simulink model "IVR"  (R2017b)
settings: Solver=VariableStepAuto  StartTime=0.0  StopTime=4e-06  MaxStep=1e-09  MinStep=1e-13  RelTol=1e-3
values from neighbouring files (symbols this model uses):
  ADC_reso = (ADC_higher_range-ADC_lower_range)/2^ADC_reso_bits    [ivr_specs_gen.m]
  DPWM_reso = (DPWM_upper_limit-DPWM_lower_limit)/2^DPWM_reso_bits    [ivr_specs_gen.m]
libraries: simulink x1, powerlib_meascontrol x1
settings Model: Creator=ndasari3  LastModifiedBy=nihar
settings CodeAppCC: StateflowObjectComments=on
settings SimscapeCC: SimscapeNormalizeSystem=off

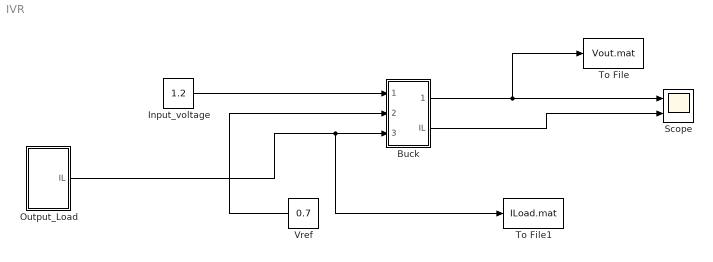
== system IVR ==
  Buck : Subsystem
  Input_voltage : Constant  Value=1.2
  Output_Load : Subsystem
  Scope : Scope  NumInputPorts=2
  To File : ToFile  Filename=Vout.mat  MatrixName=Vout  SaveFormat=Timeseries
  To File1 : ToFile  Filename=ILoad.mat  MatrixName=ILoad  SaveFormat=Timeseries
  Vref : Constant  Value=0.7
  wires:
  Input_voltage/1 -> Buck/1(Vin)
  Vref/1 -> Buck/2(Vref)
  Output_Load/1(IL) -> To File1/1, Buck/3(Iout)
  Buck/1(Vout) -> To File/1, Scope/1
  Buck/2(IL) -> Scope/2

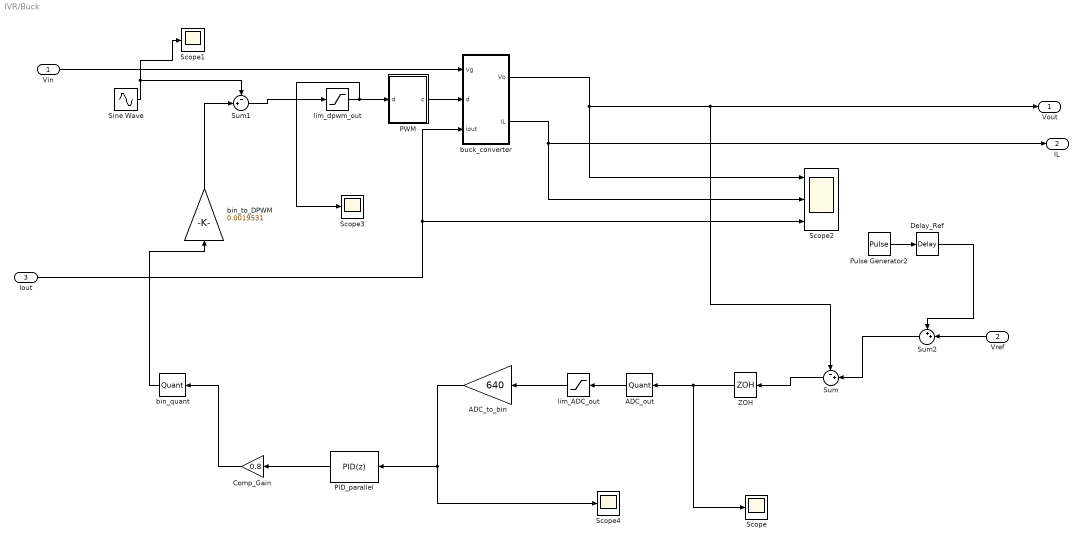
== system IVR/Buck ==
  Vin : Inport
  Vref : Inport  Port=2
  Iout : Inport  Port=3
  ADC_out : Quantizer  QuantizationInterval=0.0015625
  ADC_to_bin : Gain  Gain=640  RndMeth=Nearest
  Comp_Gain : Gain  Gain=0.8
  Delay_Ref : TransportDelay  DelayTime=0  BufferSize=64512
  PID_parallel : simulink/Continuous/PID Controller  Controller=PID  TimeDomain=Discrete-time  SampleTime=4e-09  IntegratorMethod=Backward Euler  FilterMethod=Forward Euler  Form=Parallel  UseFilter=off  ControllerParametersSource=internal  P=1.338  I=10436585.834  D=3.7629e-09  N=100  InitialConditionSource=internal  InitialConditionForIntegrator=0  InitialConditionForFilter=0  ExternalReset=none  LimitOutput=on  UpperSaturationLimit=1/ADC_reso  LowerSaturationLimit=0  LinearizeAsGain=off  AntiWindupMode=none  Kb=1  TrackingMode=off  Kt=1  PParamMin=[]  PParamMax=[]  IParamMin=[]  IParamMax=[]  DParamMin=[]  DParamMax=[]  NParamMin=[]  NParamMax=[]  KbParamMin=[]  KbParamMax=[]  KtParamMin=[]  KtParamMax=[]  POutMin=[]  POutMax=[]  IOutMin=[]  IOutMax=[]  DOutMin=[]  DOutMax=[]  NOutMin=[]  NOutMax=[]  KbOutMin=[]  KbOutMax=[]  KtOutMin=[]  KtOutMax=[]  IntegratorOutMin=[]  IntegratorOutMax=[]  FilterOutMin=[]  FilterOutMax=[]  SumOutMin=[]  SumOutMax=[]  SumI1OutMin=[]  SumI1OutMax=[]  SumI2OutMin=[]  SumI2OutMax=[]  SumI3OutMin=[]  SumI3OutMax=[]  SumDOutMin=[]  SumDOutMax=[]  SaturationOutMin=[]  SaturationOutMax=[]  IntegratorContinuousStateAttributes=''  IntegratorStateMustResolveToSignalObject=off  IntegratorRTWStateStorageClass=Auto  FilterContinuousStateAttributes=''  FilterStateMustResolveToSignalObject=off  FilterRTWStateStorageClass=Auto  DifferentiatorICPrevScaledInput=0  DifferentiatorOutMin=[]  DifferentiatorOutMax=[]  InitialConditionSetting=State (most efficient)  FilterDiffOutCoefMin=[]  FilterDiffOutCoefMax=[]  SumDenOutMin=[]  SumDenOutMax=[]  SumNumOutMin=[]  SumNumOutMax=[]  ReciprocalOutMin=[]  ReciprocalOutMax=[]  DivideOutMin=[]  DivideOutMax=[]  TunerSelectOption=Transfer Function Based (PID Tuner App)
  PWM : Subsystem
  Pulse Generator2 : DiscretePulseGenerator  PulseType=Time based  Amplitude=0  Period=1e-6  PulseWidth=50  PhaseDelay=5e-6
  Scope{,1,3..4} (4 alike) : Scope
  Scope2 : Scope  NumInputPorts=3
  Sine Wave : Sin  SineType=Sample based  Amplitude=DPWM_reso/4  Bias=DPWM_reso/4  Frequency=2*pi*125e6  Samples=3  SampleTime=4e-9
  Sum : Sum  Inputs=-+|  SaturateOnIntegerOverflow=on  InputSameDT=on  OutDataTypeStr=Inherit: Same as first input
  Sum1 : Sum  Inputs=-+|  SaturateOnIntegerOverflow=on  InputSameDT=on  OutDataTypeStr=Inherit: Same as first input
  Sum2 : Sum  Inputs=++|  SaturateOnIntegerOverflow=on  InputSameDT=on  OutDataTypeStr=Inherit: Same as first input
  ZOH : ZeroOrderHold  SampleTime=4e-09
  bin_quant : Quantizer  QuantizationInterval=1
  bin_to_DPWM : Gain  Gain=0.0019531
  buck_converter : Subsystem
  lim_ADC_out : Saturate  UpperLimit=0.2  LowerLimit=-0.2  ZeroCross=off
  lim_dpwm_out : Saturate  UpperLimit=1  LowerLimit=0
  Vout : Outport
  IL : Outport  Port=2
  wires:
  Vin/1 -> buck_converter/1(Vg)
  Vref/1 -> Sum2/2
  Iout/1 -> buck_converter/3(iout), Scope2/3
  Pulse Generator2/1 -> Delay_Ref/1
  Delay_Ref/1 -> Sum2/1
  Sum2/1 -> Sum/2
  Comp_Gain/1 -> bin_quant/1
  ADC_out/1 -> lim_ADC_out/1
  bin_quant/1 -> bin_to_DPWM/1
  lim_ADC_out/1 -> ADC_to_bin/1
  ADC_to_bin/1 -> PID_parallel/1, Scope4/1
  buck_converter/1(Vo) -> Sum/1, Vout/1, Scope2/1
  lim_dpwm_out/1 -> Scope3/1, PWM/1(d)
  Sum/1 -> ZOH/1
  buck_converter/2(IL) -> IL/1, Scope2/2
  ZOH/1 -> Scope/1, ADC_out/1
  bin_to_DPWM/1 -> Sum1/2
  PWM/1(c) -> buck_converter/2(d)
  Sine Wave/1 -> Sum1/1, Scope1/1
  Sum1/1 -> lim_dpwm_out/1
  PID_parallel/1 -> Comp_Gain/1

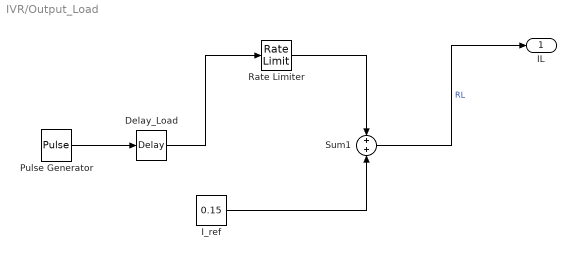
== system IVR/Output_Load ==
  Delay_Load : TransportDelay  DelayTime=2e-06  BufferSize=64512
  I_ref : Constant  Value=0.15
  Pulse Generator : DiscretePulseGenerator  PulseType=Time based  Amplitude=0.25  Period=1  PulseWidth=50
  Rate Limiter : RateLimiter  RisingSlewLimit=1/1e-9  FallingSlewLimit=-1/1e-9  SampleTimeMode=inherited
  Sum1 : Sum  Inputs=+|+  SaturateOnIntegerOverflow=on  InputSameDT=on  OutDataTypeStr=Inherit: Same as first input
  IL : Outport
  wires:
  Delay_Load/1 -> Rate Limiter/1
  Sum1/1 -> IL/1  "RL"
  I_ref/1 -> Sum1/2
  Pulse Generator/1 -> Delay_Load/1
  Rate Limiter/1 -> Sum1/1

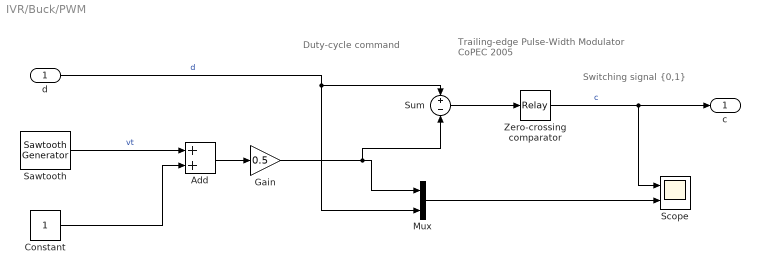
== system IVR/Buck/PWM ==
  note: Duty-cycle
      | command
  note: Switching signal {0,1}
  note: Trailing-edge Pulse-Width Modulator
      | CoPEC 2005
  d : Inport
  Add : Sum
  Constant : Constant
  Gain : Gain  Gain=0.5
  Mux : Mux  Inputs=2
  Sawtooth : powerlib_meascontrol/Pulse & Signal Generators/Sawtooth Generator  Freq=125000000  Phase=0  Ts=0
      settings: SourceProductName=Simscape Power Systems
  Scope : Scope  NumInputPorts=2
  Sum : Sum  Inputs=+|-  SaturateOnIntegerOverflow=on  InputSameDT=on  OutDataTypeStr=Inherit: Same as first input
  Zero-crossing comparator : Relay  OnSwitchValue=0.01  OffSwitchValue=-0.01
  c : Outport
  wires:
  d/1 -> Mux/2, Sum/1  "d"
  Zero-crossing comparator/1 -> c/1, Scope/1  "c"
  Sum/1 -> Zero-crossing comparator/1
  Mux/1 -> Scope/2
  Sawtooth/1 -> Add/1  "vt"
  Constant/1 -> Add/2
  Add/1 -> Gain/1
  Gain/1 -> Sum/2, Mux/1

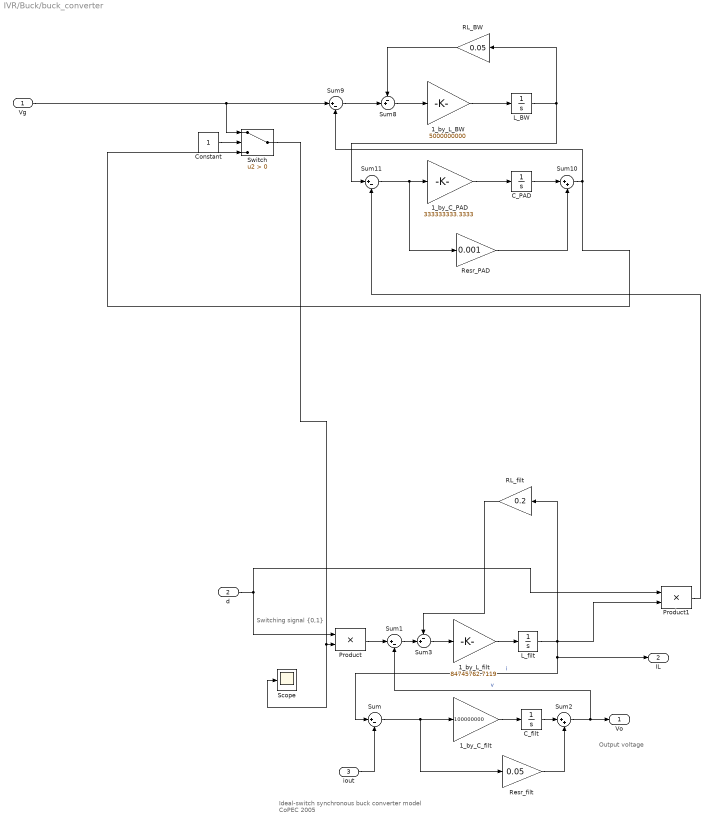
== system IVR/Buck/buck_converter ==
  note: Output voltage
  note: Switching signal {0,1}
  note: Ideal-switch synchronous buck converter model
      | CoPEC 2005
  Vg : Inport
  d : Inport  Port=2
  iout : Inport  Port=3
  1_by_C_PAD : Gain  Gain=333333333.3333  SaturateOnIntegerOverflow=on  OutDataTypeStr=Inherit: Same as input  ParamDataTypeStr=Inherit: Same as input
  1_by_C_filt : Gain  Gain=100000000  SaturateOnIntegerOverflow=on  OutDataTypeStr=Inherit: Same as input  ParamDataTypeStr=Inherit: Same as input
  1_by_L_BW : Gain  Gain=5000000000  SaturateOnIntegerOverflow=on  OutDataTypeStr=Inherit: Same as input  ParamDataTypeStr=Inherit: Same as input
  1_by_L_filt : Gain  Gain=84745762.7119  SaturateOnIntegerOverflow=on  OutDataTypeStr=Inherit: Same as input  ParamDataTypeStr=Inherit: Same as input
  C_PAD : Integrator
  C_filt : Integrator  InitialCondition=1
  Constant : Constant
  L_BW : Integrator
  L_filt : Integrator
  Product : Product  SaturateOnIntegerOverflow=on  RndMeth=Zero  InputSameDT=on  OutDataTypeStr=Inherit: Same as first input
  Product1 : Product  SaturateOnIntegerOverflow=on  RndMeth=Zero  InputSameDT=on  OutDataTypeStr=Inherit: Same as first input
  RL_BW : Gain  Gain=0.05  SaturateOnIntegerOverflow=on  OutDataTypeStr=Inherit: Same as input  ParamDataTypeStr=Inherit: Same as input
  RL_filt : Gain  Gain=0.2  SaturateOnIntegerOverflow=on  OutDataTypeStr=Inherit: Same as input  ParamDataTypeStr=Inherit: Same as input
  Resr_PAD : Gain  Gain=0.001  SaturateOnIntegerOverflow=on  OutDataTypeStr=Inherit: Same as input  ParamDataTypeStr=Inherit: Same as input
  Resr_filt : Gain  Gain=0.05  SaturateOnIntegerOverflow=on  OutDataTypeStr=Inherit: Same as input  ParamDataTypeStr=Inherit: Same as input
  Scope : Scope
  Sum{,1,9,11} (4 alike) : Sum  Inputs=|+-  SaturateOnIntegerOverflow=on  InputSameDT=on  OutDataTypeStr=Inherit: Same as first input
  Sum10 : Sum  Inputs=|++  SaturateOnIntegerOverflow=on  InputSameDT=on  OutDataTypeStr=Inherit: Same as first input
  Sum2 : Sum  Inputs=|++  SaturateOnIntegerOverflow=on  InputSameDT=on  OutDataTypeStr=Inherit: Same as first input
  Sum3 : Sum  Inputs=-+|  SaturateOnIntegerOverflow=on  InputSameDT=on  OutDataTypeStr=Inherit: Same as first input
  Sum8 : Sum  Inputs=-+|  SaturateOnIntegerOverflow=on  InputSameDT=on  OutDataTypeStr=Inherit: Same as first input
  Switch : Switch  Criteria=u2 > Threshold
  Vo : Outport
  IL : Outport  Port=2
  wires:
  Resr_filt/1 -> Sum2/2
  C_filt/1 -> Sum2/1
  Sum3/1 -> 1_by_L_filt/1
  Sum1/1 -> Sum3/2
  Sum2/1 -> Sum1/2, Vo/1  "v"
  Product/1 -> Sum1/1
  L_filt/1 -> IL/1, Sum/1, RL_filt/1, Product1/2  "i"
  1_by_L_filt/1 -> L_filt/1
  Sum/1 -> 1_by_C_filt/1, Resr_filt/1
  1_by_C_filt/1 -> C_filt/1
  Sum10/1 -> Switch/3, Sum9/2
  L_BW/1 -> RL_BW/1, Sum11/1
  1_by_L_BW/1 -> L_BW/1
  Sum8/1 -> 1_by_L_BW/1
  RL_BW/1 -> Sum8/1
  Sum9/1 -> Sum8/2
  1_by_C_PAD/1 -> C_PAD/1
  C_PAD/1 -> Sum10/1
  Sum11/1 -> Resr_PAD/1, 1_by_C_PAD/1
  Resr_PAD/1 -> Sum10/2
  Product1/1 -> Sum11/2
  iout/1 -> Sum/2
  d/1 -> Product/1, Product1/1
  Switch/1 -> Scope/1, Product/2
  Vg/1 -> Switch/1, Sum9/1
  Constant/1 -> Switch/2
  RL_filt/1 -> Sum3/1
